simulink model "macfir_hw_w_frames_tb"  (Simulink 7.6)
settings: Solver=ode3  SolverMode=SingleTasking  StartTime=0.0  StopTime=Inf  RelTol=1e-3
libraries: xbsIndex_r4 x3, simulink x2, xbsCopyrightNotice_r4 x1
settings Model: Creator=alexc  LastModifiedBy=douangp
settings DataIOCC: SignalLoggingName=sigsOut
settings OptimizationCC: InlineInvariantSignals=on  InitFltsAndDblsToZero=on
settings DebuggingCC: SaveWithParameterizedLinksMsg=none  SignalResolutionControl=TryResolveAllWithWarning  SolverPrmCheckMsg=none  MultiTaskDSMMsg=warning  MultiTaskCondExecSysMsg=none  StrictBusMsg=None
settings HardwareCC: TargetUnknown=on
settings RTWCC: IncludeERTFirstTime=on
settings GRTTargetCC: TargetFcnLib=ansi_tfl_tmw.mat

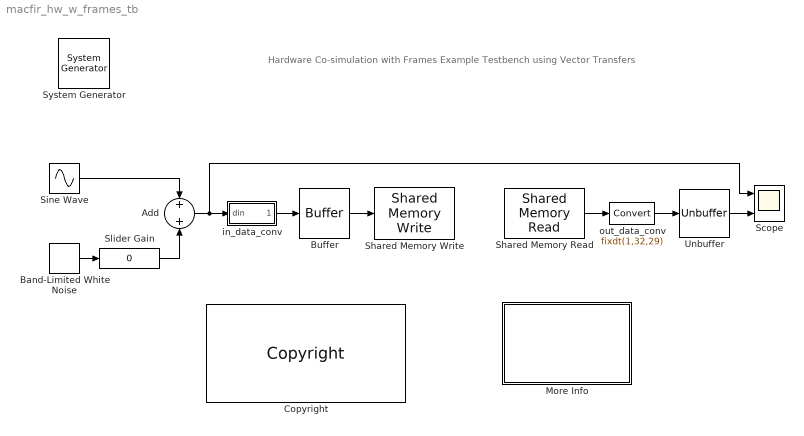
== system macfir_hw_w_frames_tb ==
  note: Hardware Co-simulation with Frames Example Testbench
      | using Vector Transfers
  " System Generator" : xbsIndex_r4/ System Generator  Tag=genX  SystemSampleTime=-1  xilinxfamily=kintex7  part=xc7k325t  speed=-1  package=ffg900  synthesis_tool=XST  clock_wrapper=Clock Enables  directory=./netlist  proj_type=Project Navigator  Synth_file=XST Defaults  Impl_file=ISE Defaults  testbench=off  simulink_period=1  sysclk_period=100  dcm_input_clock_period=10  incr_netlist=off  trim_vbits=Everywhere in SubSystem  dbl_ovrd=According to Block Masks  core_generation=According to Block Masks  run_coregen=off  deprecated_control=off  eval_field=0  block_type=sysgen
      settings: block_version=11.1.2
  Add : Sum
  Band-Limited White Noise : simulink/Sources/Band-Limited White Noise  SystemSampleTime=-1  Cov=[0.01]  Ts=1  seed=[23341]
  Buffer : Buffer  N=4095
  Copyright : xbsCopyrightNotice_r4/Copyright  copyrighttext="Copyright (c) 2011  by  Xilinx, Inc. All rights reserved.<br><br>This file contains proprietary, confidential information of Xilinx, Inc., is distributed under license from Xilinx, Inc., and may be used, copied and/or disclosed only pursuant to the terms of a valid license agreement with Xilinx, Inc. Xilinx hereby grants you a license to use this file solely for design, simulation, implementation and creation of design files limited to Xilinx devices or technologies. Use with non-Xilinx devices or technologies is expressly prohibited and immediately terminates your license unless covered by a separate agreement.<br><br>Xilinx is providing this design, code, or information \"as-is\" solely for use in developing programs and solutions for Xilinx devices, with no obligation on the part of Xilinx to provide support. By providing this design, code, or information as one possible implementation of this feature, application or standard, Xilinx is making no representation that this implementation is free from any claims of infringement. You are responsible for obtaining any rights you may require for your implementation. Xilinx expressly disclaims any warranty whatsoever with respect to the adequacy of the implementation, including but not limited to any warranties or representations that this implementation is free from claims of infringement, implied warranties of merchantability or fitness for a particular purpose.<br><br>Xilinx products are not intended for use in life support appliances, devices, or systems. Use in such applications is expressly prohibited.<br><br>Any modifications that are made to the Source Code are done at the user's sole risk and will be unsupported.<br><br>This copyright and support notice must be retained as part of this text at all times. (c) Copyright 1995-2011 Xilinx, Inc. All rights reserved."  block_type=copyright
      settings: block_version=11.1.2
  More Info : Subsystem
      mask Display: disp('Double click\n for\n more information.')
  Scope : Scope  NumInputPorts=2
      settings: TimeRange=10000  YMin=-1~-2  YMax=1~2
  Shared Memory Read : xbsIndex_r4/Shared Memory Read  Priority=20  shmem_name='VA'  shmem_type=FIFO  sample_time=4095  dataType=int32  outDims=[4095 1]  isFrame=on  shmem_word=32  shmem_depth=4095  block_type=fromshmem
      settings: AttributesFormatString=<< %<shmem_name> >>  infoedit=Reads sequentially from a shared memory block.  block_version=VER_STRING_GOES_HERE
  Shared Memory Write : xbsIndex_r4/Shared Memory Write  Priority=2  shmem_name='CA'  shmem_type=FIFO  skip_check=on  shmem_word=16  shmem_depth=4095  block_type=toshmem
      settings: AttributesFormatString=<< %<shmem_name> >>  infoedit=Writes scalar, vector, matrix, or frame data into a shared memory.  block_version=VER_STRING_GOES_HERE
  Sine Wave : Sin  Frequency=1/(10*pi)  SampleTime=1
  Slider Gain : simulink/Math Operations/Slider Gain  SystemSampleTime=-1  low=0  gain=0  high=10
  Unbuffer : Unbuffer
  in_data_conv : Subsystem
  out_data_conv : DataTypeConversion  OutDataTypeStr=fixdt(1,32,29)  ConvertRealWorld=Stored Integer (SI)  RndMeth=Nearest
  wires:
  Add/1 -> Scope/1, in_data_conv/1(din)
  Buffer/1 -> Shared Memory Write/1
  in_data_conv/1(dout) -> Buffer/1
  out_data_conv/1 -> Unbuffer/1
  Shared Memory Read/1 -> out_data_conv/1
  Unbuffer/1 -> Scope/2
  Sine Wave/1 -> Add/1
  Band-Limited White Noise/1 -> Slider Gain/1
  Slider Gain/1 -> Add/2

== system macfir_hw_w_frames_tb/More Info ==
  note: This design implements the testbench for the  32-tap MAC FIR filter that removes the additive white noise
      | from a sinusoid input source. In this testbench a Simulink Buffer block builds a frame of scalar input samples
      | by sequentially buffering the unfiltered input data.
      |
      | Please refer to the 'Using Vector Transfers' section in the System Generator for DSP User Guide
  note: Hardware Co-simulation with Frames Example Testbench
      | using Vector Transfers

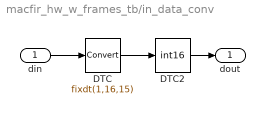
== system macfir_hw_w_frames_tb/in_data_conv ==
  din : Inport
  DTC : DataTypeConversion  OutDataTypeStr=fixdt(1,16,15)  RndMeth=Nearest  SaturateOnIntegerOverflow=on
  DTC2 : DataTypeConversion  OutDataTypeStr=int16  ConvertRealWorld=Stored Integer (SI)  RndMeth=Nearest
  dout : Outport
  wires:
  DTC/1 -> DTC2/1
  din/1 -> DTC/1
  DTC2/1 -> dout/1
